simulink model "Pid"  (R2020b)
settings: Solver=VariableStepAuto  StartTime=0.0  StopTime=10.0  RelTol=1e-3
model workspace (MAT data in the model file):
  Kd = Simulink.Parameter
  Kd.Value = 0.489767517466
  Kd.DataType = 'auto'
  Kd.Dimensions = [1 1]
  Ki = Simulink.Parameter
  Ki.Value = 4810.143607
  Ki.DataType = 'auto'
  Ki.Dimensions = [1 1]
  Kp = Simulink.Parameter
  Kp.Value = 97.1186
  Kp.DataType = 'auto'
  Kp.Dimensions = [1 1]
  N = Simulink.Parameter
  N.Value = 119827.875341
  N.DataType = 'auto'
  N.Dimensions = [1 1]
settings Model: DataDictionary=pid_data_dictionary.sldd  Creator=Lenovo  LastModifiedBy=Lenovo

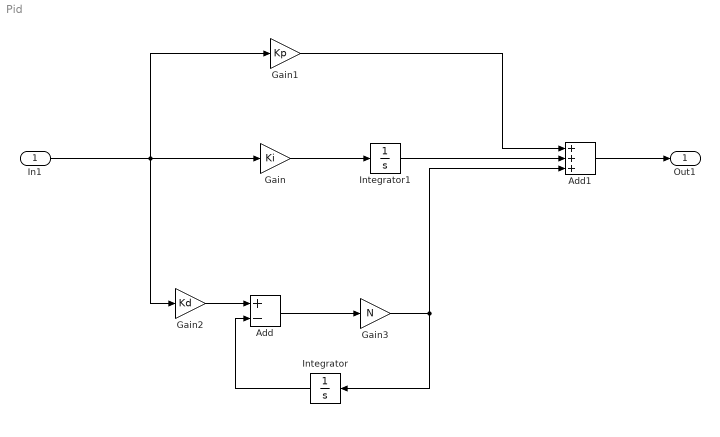
== system Pid ==
  In1 : Inport
  Add : Sum  Inputs=+-
  Add1 : Sum  Inputs=+++
  Gain : Gain  Gain=Ki
  Gain1 : Gain  Gain=Kp
  Gain2 : Gain  Gain=Kd
  Gain3 : Gain  Gain=N
  Integrator : Integrator
  Integrator1 : Integrator
  Out1 : Outport
  wires:
  In1/1 -> Gain1/1, Gain/1, Gain2/1
  Gain2/1 -> Add/1
  Add/1 -> Gain3/1
  Gain3/1 -> Add1/3, Integrator/1
  Gain/1 -> Integrator1/1
  Integrator1/1 -> Add1/2
  Integrator/1 -> Add/2
  Gain1/1 -> Add1/1
  Add1/1 -> Out1/1
